simulink library "Power_FuelCell1Motor"  (R2019b)
settings: Solver=VariableStepAuto  StartTime=0.0  StopTime=10.0  RelTol=1e-3
undefined symbols (not defined in the file or in its folder): Init, Powertrain
libraries: fl_lib x84, nesl_utility x29, GasN_lib x21, SimscapeFluids_lib x6, simulink_extras x5, customMath_lib x5, ee_lib x3, gn_supplement_lib x2, simulink x2, custom_dcdc_uni_lib x1, sm_lib x1
(part 1 of 2)
Description:
  | Component of Simscape Vehicle Templates Library
  | 
  | Copyright 2018-2020 The MathWorks, Inc.
settings Model: Creator=smiller  LastModifiedBy=smiller
settings DataIOCC: ReturnWorkspaceOutputs=off
settings DebuggingCC: ArithmeticOperatorsInVariantConditions=warning
settings SFSimCC: CustomCodeUndefinedFunction=UseInterfaceOnly

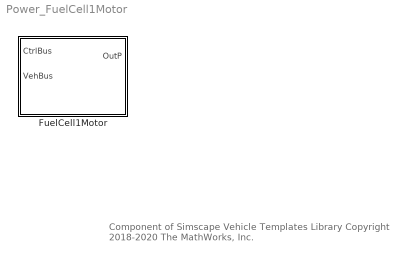
== system Power_FuelCell1Motor ==
  note: Component of Simscape Vehicle Templates Library
      | Copyright 2018-2020 The MathWorks, Inc.
  FuelCell1Motor : Subsystem  mask{Power=Powertrain.Power}
      mask prompts: Power "Power (structure)"
      mask Display: image('sm_car_vehicle_power_fc1motor_IMAGE.png');

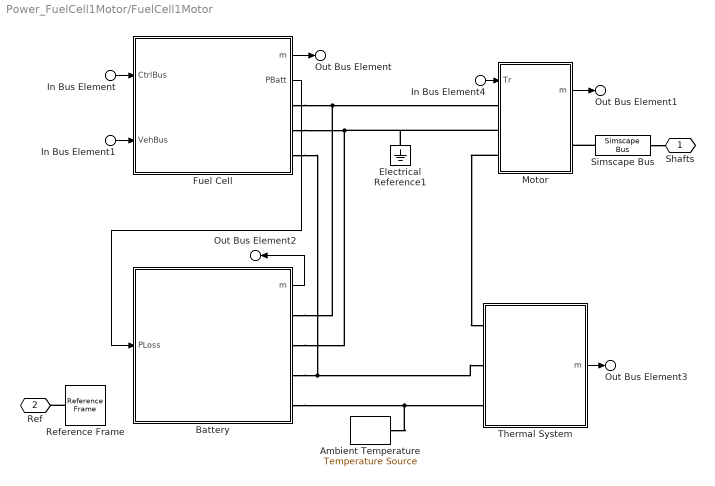
== system Power_FuelCell1Motor/FuelCell1Motor ==
  In Bus Element : Inport  PortName=CtrlBus  Element=FuelCell
  In Bus Element4 : Inport  PortName=CtrlBus  Element=Motor.trqCmd
  In Bus Element1 : Inport  Port=2  PortName=VehBus  Element=Body.CG
  Ambient Temperature : fl_lib/Thermal/Thermal Sources/Temperature Source  temperature=300 K
      settings: SourceProductName=Simscape
  Battery : Subsystem  VariantControl=0  mask{Battery=Power.Battery}
      mask prompts: Battery "Battery (structure)"
      mask Display: image('sm_car_vehicle_power_battery_system_IMAGE.png');
  Electrical Reference1 : fl_lib/Electrical/Electrical Elements/Electrical Reference
  Fuel Cell : Subsystem  VariantControl=0  mask{FuelCell=Power.FuelCell}
      mask prompts: FuelCell "Fuel Cell (structure)"
      mask Display: image('sm_car_vehicle_power_fuel_cell_converter_IMAGE.png');
  Motor : Subsystem  mask{Motor=Power.MotorF}
      mask prompts: Motor "Motor (structure)"
      mask Display: image('sm_car_vehicle_power_emotor_simplified_IMAGE.png');
  Reference Frame : sm_lib/Frames and Transforms/Reference Frame
  Simscape Bus : SimscapeBus  HierarchyStrings=ShaftF
  Thermal System : Subsystem  mask{Cooling=Power.Cooling}
      mask prompts: Cooling "Cooling (structure)"
      mask Display: image('sm_car_vehicle_power_cooling_active1loop_IMAGE.png');
  Shafts : PMIOPort  Side=Left
  Ref : PMIOPort  Port=2  Side=Right
  Out Bus Element : Outport  PortName=OutP  Element=FuelCell
  Out Bus Element1 : Outport  PortName=OutP  Element=Motor
  Out Bus Element2 : Outport  PortName=OutP  Element=Battery
  Out Bus Element3 : Outport  PortName=OutP  Element=Thermal
  wires:
  Fuel Cell/2(PBatt) -> Battery/1(PLoss)
  In Bus Element/1 -> Fuel Cell/1(CtrlBus)
  In Bus Element4/1 -> Motor/1(Tr)
  In Bus Element1/1 -> Fuel Cell/2(VehBus)
  Motor/1(m) -> Out Bus Element1/1
  Fuel Cell/1(m) -> Out Bus Element/1
  Thermal System/1(m) -> Out Bus Element3/1
  Battery/1(m) -> Out Bus Element2/1
  connections:
  Simscape Bus/LConn1 -- Motor/RConn1
  Battery/RConn2 -- Motor/LConn2 -- Electrical Reference1/LConn1 -- Fuel Cell/RConn2
  Simscape Bus/RConn1 -- Shafts/RConn1
  Motor/LConn3 -- Thermal System/LConn1
  Battery/RConn3 -- Fuel Cell/RConn3 -- Thermal System/LConn2
  Ambient Temperature/LConn1 -- Battery/RConn4 -- Thermal System/LConn3
  Battery/RConn1 -- Fuel Cell/RConn1 -- Motor/LConn1
  Reference Frame/RConn1 -- Ref/RConn1

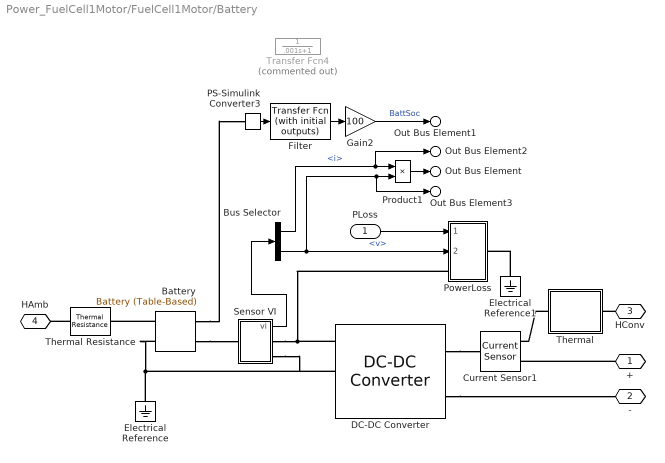
== system Power_FuelCell1Motor/FuelCell1Motor/Battery ==
  PLoss : Inport
  Battery : ee_lib/Sources/Battery (Table-Based)  SOC_vec=Battery.vNoLoad.SOC.Value  T_dependence=ee.enum.temperature_dependence.yes  T_vec=Battery.vNoLoad.T.Value K  V0_mat=Battery.vNoLoad.V0.Value V  V0_vec=[3.1, 3.27, 3.31, 3.5] V  R0_mat=Battery.rTerminal.R0.Value Ohm  R0_vec=[.015, .017, .012, .013] Ohm  AH_vec=Battery.AhTable.Ah.Value hr*A  AH=4.1 hr*A  prm_leak=1  Rleak_vec=ones(size(Battery.vNoLoad.T.Value))*10000 Ohm  Rleak=7e3 Ohm  prm_dyn=1  R1_mat=[.089, .076, .01; .042, .022, .099; .019, .007, .002; .051, .043, .029] Ohm  R1_vec=[.076, .022, .007, .043] Ohm  tau1_mat=[44, 148, 235; 93, 110, 1000; 19, 27, 133; .5, 22, 3] s  tau1_vec=[148, 110, 27, 22] s  R2_mat=[.014, .382, .407; .028, .006, .007; .014, .007, .006; .333, .956, .912] Ohm  R2_vec=[.382, .006, .007, .956] Ohm  tau2_mat=[1, 44, 5644; 11, 24, 506; 2, 14, 330; 3310, 13419, 30216] s  tau2_vec=[44, 24, 14, 13419] s  R3_mat=[.014, .382, .407; .028, .006, .007; .014, .007, .006; .333, .956, .912] Ohm  R3_vec=[.382, .006, .007, .956] Ohm  tau3_mat=[1, 44, 5644; 11, 24, 506; 2, 14, 330; 3310, 13419, 30216] s  tau3_vec=[44, 24, 14, 13419] s  R4_mat=[.014, .382, .407; .028, .006, .007; .014, .007, .006; .333, .956, .912] Ohm  R4_vec=[.382, .006, .007, .956] Ohm  tau4_mat=[1, 44, 5644; 11, 24, 506; 2, 14, 330; 3310, 13419, 30216] s  tau4_vec=[44, 24, 14, 13419] s  R5_mat=[.014, .382, .407; .028, .006, .007; .014, .007, .006; .333, .956, .912] Ohm  R5_vec=[.382, .006, .007, .956] Ohm  tau5_mat=[1, 44, 5644; 11, 24, 506; 2, 14, 330; 3310, 13419, 30216] s  tau5_vec=[44, 24, 14, 13419] s  prm_fade=ee.enum.battery.prm_fade.equations  N0=100  dV0=0  dR0=0  dAH=0  dRleak=0  dR1=0  dR2=0  dR3=0  dR4=0  dR5=0  N0vec=[100, 200, 300]  Tfadevec=[298.15, 323.15] K  dV0vec=[0, 0, 0]  dR0vec=[0, 0, 0]  dAHvec=[0, 0, 0]  dRleakvec=[0, 0, 0]  dR1vec=[0, 0, 0]  dR2vec=[0, 0, 0]  dR3vec=[0, 0, 0]  dR4vec=[0, 0, 0]  dR5vec=[0, 0, 0]  dV0mat=[0, 0; 0, 0; 0, 0]  dR0mat=[0, 0; 0, 0; 0, 0]  dAHmat=[0, 0; 0, 0; 0, 0]  dRleakmat=[0, 0; 0, 0; 0, 0]  dR1mat=[0, 0; 0, 0; 0, 0]  dR2mat=[0, 0; 0, 0; 0, 0]  dR3mat=[0, 0; 0, 0; 0, 0]  dR4mat=[0, 0; 0, 0; 0, 0]  dR5mat=[0, 0; 0, 0; 0, 0]  temperature=Battery.TInit.Value K  i_specify=off  i_priority=None  i=0 A  i_nominal_specify=off  i_nominal_unit=A  i_nominal_value=1  v_specify=off  v_priority=None  v=0 V  v_nominal_specify=off  v_nominal_unit=V  v_nominal_value=1  stateOfCharge_specify=on  stateOfCharge_priority=High  stateOfCharge=Battery.SOCInit.Value  stateOfCharge_nominal_specify=off  stateOfCharge_nominal_unit=1  stateOfCharge_nominal_value=1  num_cycles_specify=off  num_cycles_priority=High  num_cycles=0  num_cycles_nominal_specify=off  num_cycles_nominal_unit=1  num_cycles_nominal_value=1  thermal_mass=Battery.mThermal.Value J/K  temperature_specify=on  temperature_priority=High  temperature_nominal_specify=off  temperature_nominal_unit=K  temperature_nominal_value=1
      settings: SourceProductName=Simscape Electrical  SourceProductBaseCode=PS  InternalSimscapePortConfiguration="{\"Bottom\":[],\"Left\":[{\"id\":\"p\",\"label\":\"+\",\"type\":\"foundation.electrical.electrical\"},{\"id\":\"soc\",\"label\":\"SOC\",\"type\":\"output\"}],\"Right\":[{\"id\":\"n\",\"label\":\"-\",\"type\":\"foundation.electrical.electrical\"},{\"id\":\"H\",\"label\":\"H\",\"type\":\"foundation.thermal.thermal\"}],\"Top\":[]}"
  Bus Selector : BusSelector  OutputSignals=i,v
  Current Sensor1 : fl_lib/Electrical/Electrical Sensors/Current Sensor
  DC-DC Converter : ee_lib/Semiconductors & Converters/Converters/DC-DC Converter  v_ref="Battery.Converter.vRef.Value  V"  P_rated=Battery.Converter.power.Value W  droop_param=1  droop=Battery.Converter.droopVpA.Value V/A  droop_percent=2  reversible=1  efficiency=Battery.Converter.efficiency.Value  P_fixed=Battery.Converter.lossFixed.Value W  model_dynamics=0  tau=0.02 s  v_ini=650 V  G_diode=1e-6 1/Ohm  i1_max=Battery.Converter.iMaxSupply.Value A  fault_condition=1  fault_threshold=0.5  thermal_mass=100 J/K  initial_temperature=298.15 K
      settings: SourceProductName=Simscape Electrical  SourceProductBaseCode=PS  InternalSimscapePortConfiguration="{\"Bottom\":[],\"Left\":[{\"id\":\"p1\",\"label\":\"1+\",\"type\":\"foundation.electrical.electrical\"},{\"id\":\"n1\",\"label\":\"1-\",\"type\":\"foundation.electrical.electrical\"},{\"id\":\"F\",\"label\":\"F\",\"type\":\"input\"}],\"Right\":[{\"id\":\"p2\",\"label\":\"2+\",\"type\":\"foundation.electrical.electrical\"},{\"id\":\"n2\",\"label\":\"2-\",\"type\":\"foundation.electrical.electrical\"}],\"Top\":[]}"
  Electrical Reference : fl_lib/Electrical/Electrical Elements/Electrical Reference
  Electrical Reference1 : fl_lib/Electrical/Electrical Elements/Electrical Reference
  Filter : simulink_extras/Additional Linear/Transfer Fcn (with initial outputs)  N=[1]  D=[.01 1]  Y0=Battery.SOCInit.Value  U0=0
  Gain2 : Gain  Gain=100
  PS-Simulink Converter3 : nesl_utility/PS-Simulink Converter  PhysicalDomain=network_engine_domain  SubClassName=ps_output  LeftPortType=input  RightPortType=output  PseudoPeriodic=off  Frequencies=[]  Unit=1  AffineConversion=off
  PowerLoss : Subsystem
  Product1 : Product
  Sensor VI : Subsystem
  Thermal : Subsystem
  Thermal Resistance : fl_lib/Thermal/Thermal Elements/Thermal Resistance  resistance=Battery.rThermal.Value K/W  T_specify=off  T_priority=None  T=0 K  T_nominal_specify=off  T_nominal_unit=K  T_nominal_value=1  Q_specify=off  Q_priority=None  Q=0 W  Q_nominal_specify=off  Q_nominal_unit=W  Q_nominal_value=1
      settings: SourceProductName=Simscape  SourceProductBaseCode=SS
  Transfer Fcn4 : TransferFcn  Commented=on  Denominator=[.001 1]
  + : PMIOPort  Side=Right
  - : PMIOPort  Port=2  Side=Right
  HConv : PMIOPort  Port=3  Side=Right
  HAmb : PMIOPort  Port=4  Side=Right
  Out Bus Element : Outport  PortName=m  Element=Power
  Out Bus Element1 : Outport  PortName=m  Element=SOC
  Out Bus Element2 : Outport  PortName=m  Element=i
  Out Bus Element3 : Outport  PortName=m  Element=v
  wires:
  PS-Simulink Converter3/1 -> Filter/1
  Gain2/1 -> Out Bus Element1/1  "BattSoc"
  Filter/1 -> Gain2/1
  Bus Selector/2 -> Product1/2, Out Bus Element3/1, PowerLoss/2(VBatt)  "<v>"
  PLoss/1 -> PowerLoss/1(PLoss)
  Bus Selector/1 -> Product1/1, Out Bus Element2/1  "<i>"
  Product1/1 -> Out Bus Element/1
  Sensor VI/1(vi) -> Bus Selector/1
  connections:
  PowerLoss/LConn1 -- DC-DC Converter/LConn1 -- Sensor VI/RConn1
  Battery/LConn2 -- PS-Simulink Converter3/LConn1
  Battery/LConn1 -- Sensor VI/LConn1
  Electrical Reference/LConn1 -- Battery/RConn1 -- DC-DC Converter/LConn2 -- Sensor VI/RConn2
  Battery/RConn2 -- Thermal Resistance/RConn1
  +/RConn1 -- Current Sensor1/RConn2
  DC-DC Converter/RConn2 -- -/RConn1
  DC-DC Converter/RConn1 -- Current Sensor1/LConn1
  Thermal Resistance/LConn1 -- HAmb/RConn1
  Electrical Reference1/LConn1 -- PowerLoss/RConn1
  HConv/RConn1 -- Thermal/RConn1
  Thermal/LConn1 -- Current Sensor1/RConn1

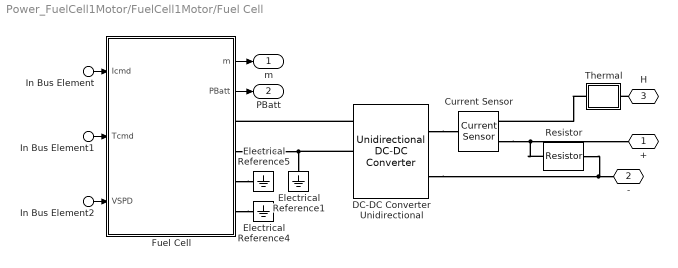
== system Power_FuelCell1Motor/FuelCell1Motor/Fuel Cell ==
  In Bus Element : Inport  PortName=CtrlBus  Element=iCmd
  In Bus Element1 : Inport  PortName=CtrlBus  Element=TFuelCellCmd
  In Bus Element2 : Inport  Port=2  PortName=VehBus  Element=vx
  Current Sensor : fl_lib/Electrical/Electrical Sensors/Current Sensor
  DC-DC Converter Unidirectional : custom_dcdc_uni_lib/Unidirectional DC-DC Converter  v_ref=FuelCell.Converter.vRef.Value V  P_rated=FuelCell.Converter.power.Value W  droop=FuelCell.Converter.droopVpA.Value V/A  efficiency=FuelCell.Converter.efficiency.Value  P_fixed=FuelCell.Converter.lossFixed.Value W  v_ini=650 V  G_diode=1e-6 1/Ohm  i1_max=FuelCell.Converter.iMaxSupply.Value A  fault_threshold=0.5
      settings: InternalSimscapePortConfiguration="{\"Bottom\":[],\"Left\":[{\"id\":\"p1\",\"label\":\"1+\",\"type\":\"foundation.electrical.electrical\"},{\"id\":\"n1\",\"label\":\"1-\",\"type\":\"foundation.electrical.electrical\"},{\"id\":\"F\",\"label\":\"F\",\"type\":\"input\"}],\"Right\":[{\"id\":\"p2\",\"label\":\"2+\",\"type\":\"foundation.electrical.electrical\"},{\"id\":\"n2\",\"label\":\"2-\",\"type\":\"foundation.electrical.electrical\"}],\"Top\":[]}"
  Electrical Reference1 : fl_lib/Electrical/Electrical Elements/Electrical Reference
  Electrical Reference4 : fl_lib/Electrical/Electrical Elements/Electrical Reference
  Electrical Reference5 : fl_lib/Electrical/Electrical Elements/Electrical Reference
  Fuel Cell : Subsystem
      mask Display: image('sm_car_vehicle_power_fuel_cell_IMAGE.png');
  Resistor : fl_lib/Electrical/Electrical Elements/Resistor  R=1e7 Ohm  i_specify=off  i_priority=None  i=0 A  i_nominal_specify=off  i_nominal_unit=A  i_nominal_value=1  v_specify=off  v_priority=None  v=0 V  v_nominal_specify=off  v_nominal_unit=V  v_nominal_value=1
  Thermal : Subsystem
  + : PMIOPort  Side=Right
  - : PMIOPort  Port=2  Side=Right
  H : PMIOPort  Port=3  Side=Right
  m : Outport
  PBatt : Outport  Port=2
  wires:
  In Bus Element2/1 -> Fuel Cell/3(VSPD)
  In Bus Element1/1 -> Fuel Cell/2(Tcmd)
  In Bus Element/1 -> Fuel Cell/1(Icmd)
  Fuel Cell/1(m) -> m/1
  Fuel Cell/2(PBatt) -> PBatt/1
  connections:
  Fuel Cell/RConn2 -- DC-DC Converter Unidirectional/LConn2 -- Electrical Reference1/LConn1
  Resistor/RConn1 -- DC-DC Converter Unidirectional/RConn2 -- -/RConn1
  Current Sensor/RConn2 -- Resistor/LConn1 -- +/RConn1
  Fuel Cell/RConn3 -- Electrical Reference5/LConn1
  Fuel Cell/RConn4 -- Electrical Reference4/LConn1
  DC-DC Converter Unidirectional/LConn1 -- Fuel Cell/RConn1
  DC-DC Converter Unidirectional/RConn1 -- Current Sensor/LConn1
  H/RConn1 -- Thermal/RConn1
  Thermal/LConn1 -- Current Sensor/RConn1

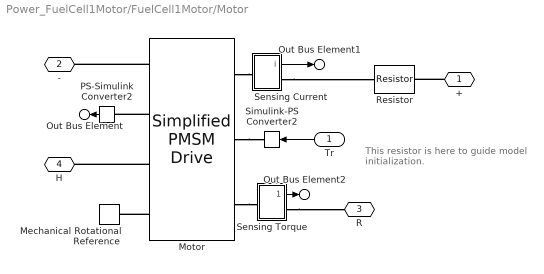
== system Power_FuelCell1Motor/FuelCell1Motor/Motor ==
  note: This resistor is here to guide model initialization.
  Tr : Inport
  Mechanical Rotational Reference : fl_lib/Mechanical/Rotational Elements/Mechanical Rotational Reference
  Motor : ee_lib/Electromechanical/Permanent Magnet/Simplified PMSM Drive  torque_speed_param=1  w_t=Motor.TorqueSpd.w.Value rpm  T_t=Motor.TorqueSpd.trq.Value N*m  torque_max=0.1 N*m  power_max=30 W  Tc=1/Motor.fActuatorCutoff.Value s  losses_param=3  eff=100  w_eff=3750 rpm  T_eff=0.08 N*m  Piron=0 W  Pbase=0 W  w_eff_vec=Motor.TorqueSpd.w.Value rpm  T_eff_vec=Motor.LossTable.trq.Value N*m  v_eff_vec=[100, 250, 400] V  losses_mat=[1.49, 1.67, 2.21, 3.1; .42, .69, 1.14, 2.03; .06, .24, .78, 1.68; .42, .69, 1.14, 2.03; 1.49, 1.67, 2.21, 3.1] W  efficiency_mat=Motor.LossTable.efficiency.Value  losses_mat_3D=ones(5, 4, 3) W  efficiency_mat_3D=95 * ones(5, 4, 3)  Res=Motor.Rsupply.Value Ohm  J=Motor.J.Value kg*m^2  lam=Motor.b.Value N*m/(rad/s)  speed0=0 rpm  faulted_specify=off  faulted_priority=None  faulted=0  faulted_nominal_specify=off  faulted_nominal_unit=1  faulted_nominal_value=1  alpha=3.93e-3 1/K  Tmeas=Motor.ThermalLoss.T1.Value degC  Tmeas2=Motor.ThermalLoss.T2.Value degC  losses_mat_T2=[1.49, 1.74, 2.49, 3.74; .42, .67, 1.42, 2.67; .06, .31, 1.06, 2.31; .42, .67, 1.42, 2.67; 1.49, 1.74, 2.49, 3.74] W  efficiency_mat_T2=Motor.ThermalLoss.efficiency.Value  losses_mat_3D_T2=ones(5, 4, 3) W  efficiency_mat_3D_T2=95 * ones(5, 4, 3)  thermal_mass=Motor.ThermalLoss.mThermal.Value J/K  initial_temperature=Motor.ThermalLoss.Tinit.Value K  fault_condition=1  fault_threshold=0.5
      settings: SourceProductName=Simscape Electrical  SourceProductBaseCode=PS  InternalSimscapePortConfiguration="{\"Bottom\":[],\"Left\":[{\"id\":\"Vp\",\"label\":\"+\",\"type\":\"foundation.electrical.electrical\"},{\"id\":\"Tr\",\"label\":\"Tr\",\"type\":\"input\"},{\"id\":\"R\",\"label\":\"R\",\"type\":\"foundation.mechanical.rotational.rotational\"}],\"Right\":[{\"id\":\"Vm\",\"label\":\"-\",\"type\":\"foundation.electrical.electrical\"},{\"id\":\"Omega\",\"label\":\"w\",\"type\":\"output\"},{\"id\":\"H\",\"label\":\"H\",\"type\":\"foundation.thermal.thermal\"},{\"id\":\"C\",\"label\":\"C\",\"type\":\"foundation.mechanical.rotational.rotational\"}],\"Top\":[]}"
  PS-Simulink Converter2 : nesl_utility/PS-Simulink Converter  PhysicalDomain=network_engine_domain  SubClassName=ps_output  LeftPortType=input  RightPortType=output  PseudoPeriodic=off  Frequencies=[]  Unit=rad/s  AffineConversion=off
  Resistor : fl_lib/Electrical/Electrical Elements/Resistor  R=1e-6 Ohm  i_specify=on  i_priority=High  i=0.1*Init.Front.nWheel.Value(1) A  i_nominal_specify=off  i_nominal_unit=A  i_nominal_value=1  v_specify=off  v_priority=None  v=0 V  v_nominal_specify=off  v_nominal_unit=V  v_nominal_value=1
  Sensing Current : Subsystem
  Sensing Torque : Subsystem
  Simulink-PS Converter2 : nesl_utility/Simulink-PS Converter  PhysicalDomain=network_engine_domain  SubClassName=ps_input  LeftPortType=input  RightPortType=output  PseudoPeriodic=off  Frequencies=[]  NoiseDistribution=none  NoiseParameters=[]  Unit=N*m  AffineConversion=off  FilteringAndDerivatives=provide  SimscapeFilterOrder=1  InputFilterTimeConstant=0.001  UdotUserProvided=0
  + : PMIOPort  Side=Left
  - : PMIOPort  Port=2  Side=Left
  R : PMIOPort  Port=3  Side=Right
  H : PMIOPort  Port=4  Side=Left
  Out Bus Element : Outport  PortName=m  Element=w
  Out Bus Element1 : Outport  PortName=m  Element=i
  Out Bus Element2 : Outport  PortName=m  Element=trq
  wires:
  PS-Simulink Converter2/1 -> Out Bus Element/1
  Tr/1 -> Simulink-PS Converter2/1
  Sensing Current/1(i) -> Out Bus Element1/1
  Sensing Torque/1(trq) -> Out Bus Element2/1
  connections:
  Motor/RConn4 -- Mechanical Rotational Reference/LConn1
  Motor/LConn2 -- Simulink-PS Converter2/RConn1
  Motor/LConn3 -- Sensing Torque/LConn1
  Motor/LConn1 -- Sensing Current/LConn1
  Motor/RConn1 -- -/RConn1
  Motor/RConn3 -- H/RConn1
  Motor/RConn2 -- PS-Simulink Converter2/LConn1
  Sensing Current/RConn1 -- Resistor/LConn1
  Sensing Torque/RConn1 -- R/RConn1
  +/RConn1 -- Resistor/RConn1

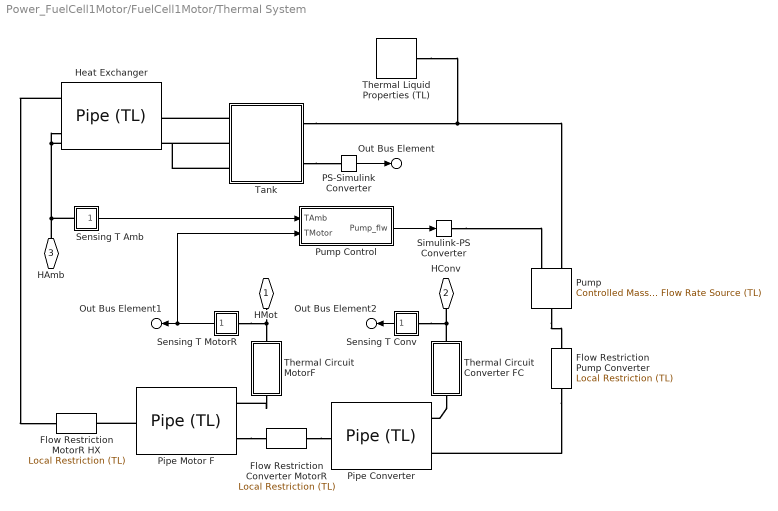
== system Power_FuelCell1Motor/FuelCell1Motor/Thermal System ==
  Flow Restriction Converter MotorR : fl_lib/Thermal Liquid/Elements/Local Restriction (TL)  restriction_type=foundation.enum.restriction_type.fixed  restriction_area=Cooling.Restriction.area.Value m^2  min_area=1e-10 m^2  max_area=0.005 m^2  area=Cooling.Restriction.areaPorts.Value m^2  Cd=Cooling.Restriction.dischargeCoeff.Value  pressure_recovery=simscape.enum.onoff.on  Re_c=Cooling.Restriction.CriticalReynolds.Value
      settings: SourceProductName=Simscape  SourceProductBaseCode=SS
  Flow Restriction MotorR HX : fl_lib/Thermal Liquid/Elements/Local Restriction (TL)  restriction_type=foundation.enum.restriction_type.fixed  restriction_area=Cooling.Restriction.area.Value m^2  min_area=1e-10 m^2  max_area=0.005 m^2  area=Cooling.Restriction.areaPorts.Value m^2  Cd=Cooling.Restriction.dischargeCoeff.Value  pressure_recovery=simscape.enum.onoff.on  Re_c=Cooling.Restriction.CriticalReynolds.Value
      settings: SourceProductName=Simscape  SourceProductBaseCode=SS
  Flow Restriction Pump Converter : fl_lib/Thermal Liquid/Elements/Local Restriction (TL)  restriction_type=foundation.enum.restriction_type.fixed  restriction_area=Cooling.Restriction.area.Value m^2  min_area=1e-10 m^2  max_area=0.005 m^2  area=Cooling.Restriction.areaPorts.Value m^2  Cd=Cooling.Restriction.dischargeCoeff.Value  pressure_recovery=simscape.enum.onoff.on  Re_c=Cooling.Restriction.CriticalReynolds.Value
      settings: SourceProductName=Simscape  SourceProductBaseCode=SS
  Heat Exchanger : SimscapeFluids_lib/Thermal Liquid/Pipes & Fittings/Pipe (TL)  dynamic_compressibility=0  inertia=0  num_segments=1  pipe_length=Cooling.HX.x.Value m  area=Cooling.HX.area.Value m^2  Dh=Cooling.HX.diameter.Value m  wall_spec=1  Dh_rigid=0.01 m  wall_compliance=1.2e-6 m/MPa  wall_time_constant=0.01 s  elevation_gain=Cooling.HX.elevation.Value m  g=9.81 m/s^2  pressure_loss_spec=1  length_add=Cooling.HX.xResistance.Value m  roughness=Cooling.HX.roughness.Value m  Re_friction_TLU=[ 400 1000 1.5e+3 3e+3 4e+3 6e+3 1e+4 2e+4 4e+4 6e+4 1e+5 1e+8 ]  friction_factor_TLU=[ 0.264 0.112 0.07099999999999999 0.0417 0.0387 0.0268 0.025 0.0232 0.0226 0.022 0.0214 0.0214 ]  shape_factor=Cooling.HX.frictionDarcy.Value  mdot_nominal=[ 0.1 1 ] kg/s  p_diff_nominal=[ 0.001 0.01 ] MPa  mdot_threshold=1e-6 kg/s  Re_lam=Cooling.HX.laminarReynoldsMax.Value  Re_tur=Cooling.HX.turbulentReynoldsMin.Value  heat_transfer_spec=1  mdot_nominal_heat=[ 0.1 1 ] kg/s  T_in_nominal=[ 293.15 293.15 ] K  T_out_nominal=[ 300 300 ] K  p_in_nominal_heat=[ 0.101325 0.101325 ] MPa  T_wall_nominal=[ 303.15 303.15 ] K  a_coeff=0.023  b_Re_power=0.8  c_Pr_power=0.4  Nu_lam=Cooling.HX.laminarNusselt.Value  Re_Colburn_TLU=[ 100 150 1000 ]  Colburn_factor_TLU=[ 0.019 0.013 0.002 ]  Re_Nu_TLU=[ 100 150 1000 ]  Pr_Nu_TLU=[ 1 10 ]  Nu_TLU=[ 3.72 4.21; 3.75 4.44; 4.21 7.15 ]  T0_vec=300 K  p0_vec=0.101325 MPa  mdot0=0.1 kg/s
      settings: SourceProductName=Simscape Fluids  SourceProductBaseCode=SH
  PS-Simulink Converter : nesl_utility/PS-Simulink Converter  PhysicalDomain=network_engine_domain  SubClassName=ps_output  LeftPortType=input  RightPortType=output  PseudoPeriodic=off  Frequencies=[]  Unit=K  AffineConversion=off
  Pipe Converter : SimscapeFluids_lib/Thermal Liquid/Pipes & Fittings/Pipe (TL)  dynamic_compressibility=0  inertia=0  num_segments=1  pipe_length=Cooling.Converter.Pipe.x.Value m  area="Cooling.Converter.Pipe.area.Value  m^2"  Dh=Cooling.Converter.Pipe.diameter.Value m  wall_spec=1  Dh_rigid=0.01 m  wall_compliance=1.2e-6 m/MPa  wall_time_constant=0.01 s  elevation_gain=Cooling.Converter.Pipe.elevation.Value m  g=9.81 m/s^2  pressure_loss_spec=1  length_add=Cooling.Converter.Pipe.xResistance.Value m  roughness=Cooling.Converter.Pipe.roughness.Value m  Re_friction_TLU=[ 400 1000 1.5e+3 3e+3 4e+3 6e+3 1e+4 2e+4 4e+4 6e+4 1e+5 1e+8 ]  friction_factor_TLU=[ 0.264 0.112 0.07099999999999999 0.0417 0.0387 0.0268 0.025 0.0232 0.0226 0.022 0.0214 0.0214 ]  shape_factor=Cooling.Converter.Pipe.frictionDarcy.Value  mdot_nominal=[ 0.1 1 ] kg/s  p_diff_nominal=[ 0.001 0.01 ] MPa  mdot_threshold=1e-6 kg/s  Re_lam=Cooling.Converter.Pipe.laminarReynoldsMax.Value  Re_tur=Cooling.Converter.Pipe.turbulentReynoldsMin.Value  heat_transfer_spec=1  mdot_nominal_heat=[ 0.1 1 ] kg/s  T_in_nominal=[ 293.15 293.15 ] K  T_out_nominal=[ 300 300 ] K  p_in_nominal_heat=[ 0.101325 0.101325 ] MPa  T_wall_nominal=[ 303.15 303.15 ] K  a_coeff=0.023  b_Re_power=0.8  c_Pr_power=0.4  Nu_lam=Cooling.Converter.Pipe.laminarNusselt.Value  Re_Colburn_TLU=[ 100 150 1000 ]  Colburn_factor_TLU=[ 0.019 0.013 0.002 ]  Re_Nu_TLU=[ 100 150 1000 ]  Pr_Nu_TLU=[ 1 10 ]  Nu_TLU=[ 3.72 4.21; 3.75 4.44; 4.21 7.15 ]  T0_vec=300 K  p0_vec=0.101325 MPa  mdot0=0.1 kg/s
      settings: SourceProductName=Simscape Fluids  SourceProductBaseCode=SH
  Pipe Motor F : SimscapeFluids_lib/Thermal Liquid/Pipes & Fittings/Pipe (TL)  dynamic_compressibility=0  inertia=0  num_segments=1  pipe_length=Cooling.MotorF.Pipe.x.Value m  area=Cooling.MotorF.Pipe.area.Value m^2  Dh=Cooling.MotorF.Pipe.diameter.Value m  wall_spec=1  Dh_rigid=0.01 m  wall_compliance=1.2e-6 m/MPa  wall_time_constant=0.01 s  elevation_gain=Cooling.MotorF.Pipe.elevation.Value m  g=9.81 m/s^2  pressure_loss_spec=1  length_add=Cooling.MotorF.Pipe.xResistance.Value m  roughness=Cooling.MotorF.Pipe.roughness.Value m  Re_friction_TLU=[ 400 1000 1.5e+3 3e+3 4e+3 6e+3 1e+4 2e+4 4e+4 6e+4 1e+5 1e+8 ]  friction_factor_TLU=[ 0.264 0.112 0.07099999999999999 0.0417 0.0387 0.0268 0.025 0.0232 0.0226 0.022 0.0214 0.0214 ]  shape_factor=Cooling.MotorF.Pipe.frictionDarcy.Value  mdot_nominal=[ 0.1 1 ] kg/s  p_diff_nominal=[ 0.001 0.01 ] MPa  mdot_threshold=1e-6 kg/s  Re_lam=Cooling.MotorF.Pipe.laminarReynoldsMax.Value  Re_tur=Cooling.MotorF.Pipe.turbulentReynoldsMin.Value  heat_transfer_spec=1  mdot_nominal_heat=[ 0.1 1 ] kg/s  T_in_nominal=[ 293.15 293.15 ] K  T_out_nominal=[ 300 300 ] K  p_in_nominal_heat=[ 0.101325 0.101325 ] MPa  T_wall_nominal=[ 303.15 303.15 ] K  a_coeff=0.023  b_Re_power=0.8  c_Pr_power=0.4  Nu_lam=Cooling.MotorF.Pipe.laminarNusselt.Value  Re_Colburn_TLU=[ 100 150 1000 ]  Colburn_factor_TLU=[ 0.019 0.013 0.002 ]  Re_Nu_TLU=[ 100 150 1000 ]  Pr_Nu_TLU=[ 1 10 ]  Nu_TLU=[ 3.72 4.21; 3.75 4.44; 4.21 7.15 ]  T0_vec=300 K  p0_vec=0.101325 MPa  mdot0=0.1 kg/s
      settings: SourceProductName=Simscape Fluids  SourceProductBaseCode=SH
  Pump : fl_lib/Thermal Liquid/Sources/Controlled Mass Flow Rate Source (TL)  area=Cooling.Pump.area.Value m^2
      settings: SourceProductName=Simscape  SourceProductBaseCode=SS  InternalSimscapePortConfiguration="{\"Bottom\":[],\"Left\":[{\"id\":\"A\",\"label\":\"A\",\"type\":\"foundation.thermal_liquid.thermal_liquid\"},{\"id\":\"M\",\"label\":\"M\",\"type\":\"input\"}],\"Right\":[{\"id\":\"B\",\"label\":\"B\",\"type\":\"foundation.thermal_liquid.thermal_liquid\"}],\"Top\":[]}"
  Pump Control : Subsystem
  Sensing T Amb : Subsystem
  Sensing T Conv : Subsystem
  Sensing T MotorR : Subsystem
  Simulink-PS Converter : nesl_utility/Simulink-PS Converter  PhysicalDomain=network_engine_domain  SubClassName=ps_input  LeftPortType=input  RightPortType=output  PseudoPeriodic=off  Frequencies=[]  NoiseDistribution=none  NoiseParameters=[]  Unit=kg/s  AffineConversion=off  FilteringAndDerivatives=filter  SimscapeFilterOrder=1  InputFilterTimeConstant=1  UdotUserProvided=0
  Tank : Subsystem
  Thermal Circuit Converter FC : Subsystem
  Thermal Circuit MotorF : Subsystem
  Thermal Liquid Properties (TL) : SimscapeFluids_lib/Thermal Liquid/Utilities/Thermal Liquid Properties (TL)  fluid_list=fluids.thermal_liquid.utilities.enum.thermal_liquid_fluid_list.ethylene_glycol  concentration_param_EG=fluids.thermal_liquid.utilities.enum.thermal_liquid_concentration.volume_fraction  concentration_param_PG=fluids.thermal_liquid.utilities.enum.thermal_liquid_concentration.volume_fraction  c_mass_SW=3.5e-3  c_mass_EG=0.1  c_mass_PG=0.1  c_mass_GL=0.1  c_vol_EG=Cooling.Fluid.rEthyleneGlycol.Value  c_vol_PG=0.1  beta_const_EG=Cooling.Fluid.bulkModulus.Value GPa  beta_const_PG=2.1791 GPa  beta_const_GL=2.1791 GPa  p_min_EG=Cooling.Fluid.pMin.Value MPa  p_min_PG=0.01 MPa  p_min_GL=0.01 MPa  p_max_EG=Cooling.Fluid.pMax.Value MPa  p_max_PG=50 MPa  p_max_GL=50 MPa  p_atm=0.101325 MPa
      settings: SourceProductName=Simscape Fluids  SourceProductBaseCode=SH
  HMot : PMIOPort  Side=Left
  HConv : PMIOPort  Port=2  Side=Left
  HAmb : PMIOPort  Port=3  Side=Left
  Out Bus Element : Outport  PortName=m  Element=TCoolant
  Out Bus Element1 : Outport  PortName=m  Element=TMotorF
  Out Bus Element2 : Outport  PortName=m  Element=TConverter
  wires:
  Pump Control/1(Pump_flw) -> Simulink-PS Converter/1
  PS-Simulink Converter/1 -> Out Bus Element/1
  Sensing T MotorR/1(T) -> Pump Control/2(TMotor), Out Bus Element1/1
  Sensing T Amb/1(T) -> Pump Control/1(TAmb)
  Sensing T Conv/1(T) -> Out Bus Element2/1
  connections:
  Pipe Motor F/LConn1 -- Flow Restriction Converter MotorR/RConn1
  Flow Restriction Converter MotorR/LConn1 -- Pipe Converter/RConn1
  Pump/RConn1 -- Flow Restriction Pump Converter/LConn1
  Simulink-PS Converter/RConn1 -- Pump/LConn2
  Thermal Circuit MotorF/RConn1 -- Pipe Motor F/LConn2
  HAmb/RConn1 -- Sensing T Amb/LConn1 -- Tank/LConn3 -- Tank/LConn2 -- Heat Exchanger/LConn2
  Heat Exchanger/LConn1 -- Flow Restriction MotorR HX/RConn1
  Flow Restriction Pump Converter/RConn1 -- Pipe Converter/LConn1
  Pipe Motor F/RConn1 -- Flow Restriction MotorR HX/LConn1
  Tank/LConn1 -- Heat Exchanger/RConn1
  Tank/RConn1 -- Thermal Liquid Properties (TL)/RConn1 -- Pump/LConn1
  Thermal Circuit Converter FC/RConn1 -- Pipe Converter/LConn2
  HMot/RConn1 -- Thermal Circuit MotorF/LConn1 -- Sensing T MotorR/LConn1
  Tank/RConn2 -- PS-Simulink Converter/LConn1
  Thermal Circuit Converter FC/LConn1 -- Sensing T Conv/LConn1 -- HConv/RConn1

== system Power_FuelCell1Motor/FuelCell1Motor/Battery/PowerLoss ==
  PLoss : Inport
  VBatt : Inport  Port=2
  Controlled Current Source : fl_lib/Electrical/Electrical Sources/Controlled Current Source
  Divide : Product  Inputs=*/
  Saturation : Saturate  UpperLimit=inf  LowerLimit=200
  Simulink-PS Converter : nesl_utility/Simulink-PS Converter  PhysicalDomain=network_engine_domain  SubClassName=ps_input  LeftPortType=input  RightPortType=output  PseudoPeriodic=off  Frequencies=[]  NoiseDistribution=none  NoiseParameters=[]  Unit=A  AffineConversion=off  FilteringAndDerivatives=filter  SimscapeFilterOrder=1  InputFilterTimeConstant=0.001  UdotUserProvided=0
  + : PMIOPort  Side=Left
  - : PMIOPort  Port=2  Side=Right
  wires:
  VBatt/1 -> Saturation/1
  PLoss/1 -> Divide/1
  Divide/1 -> Simulink-PS Converter/1
  Saturation/1 -> Divide/2
  connections:
  -/RConn1 -- Controlled Current Source/LConn1
  +/RConn1 -- Controlled Current Source/RConn2
  Simulink-PS Converter/RConn1 -- Controlled Current Source/RConn1

== system Power_FuelCell1Motor/FuelCell1Motor/Battery/Sensor VI ==
  Bus Creator : BusCreator  Inputs=2
  Current Sensor : fl_lib/Electrical/Electrical Sensors/Current Sensor
  PS-Simulink Converter2 : nesl_utility/PS-Simulink Converter  PhysicalDomain=network_engine_domain  SubClassName=ps_output  LeftPortType=input  RightPortType=output  PseudoPeriodic=off  Frequencies=[]  Unit=1  AffineConversion=off
  PS-Simulink Converter4 : nesl_utility/PS-Simulink Converter  PhysicalDomain=network_engine_domain  SubClassName=ps_output  LeftPortType=input  RightPortType=output  PseudoPeriodic=off  Frequencies=[]  Unit=1  AffineConversion=off
  Transfer Fcn1 : TransferFcn  Denominator=[.001 1]
  Transfer Fcn5 : TransferFcn  Denominator=[.001 1]
  Voltage Sensor2 : fl_lib/Electrical/Electrical Sensors/Voltage Sensor
  + : PMIOPort  Side=Left
  - : PMIOPort  Port=2  Side=Right
  G : PMIOPort  Port=3  Side=Right
  vi : Outport
  wires:
  PS-Simulink Converter4/1 -> Transfer Fcn5/1
  PS-Simulink Converter2/1 -> Transfer Fcn1/1
  Transfer Fcn1/1 -> Bus Creator/2  "i"
  Transfer Fcn5/1 -> Bus Creator/1  "v"
  Bus Creator/1 -> vi/1
  connections:
  +/RConn1 -- Current Sensor/LConn1 -- Voltage Sensor2/LConn1
  PS-Simulink Converter4/LConn1 -- Voltage Sensor2/RConn1
  Current Sensor/RConn2 -- -/RConn1
  Voltage Sensor2/RConn2 -- G/RConn1
  Current Sensor/RConn1 -- PS-Simulink Converter2/LConn1

== system Power_FuelCell1Motor/FuelCell1Motor/Battery/Thermal ==
  Controlled Heat Flow Rate Source : fl_lib/Thermal/Thermal Sources/Controlled Heat Flow Rate Source
      settings: SourceProductName=Simscape
  PS Gain : fl_lib/Physical Signals/Functions/PS Gain  Commented=on  gain=0.001 Ohm
  PS Math Function : fl_lib/Physical Signals/Functions/PS Math Function  Commented=on  fcn_choice=foundation.enum.math_function.square
      settings: SourceProductName=Simscape  SourceProductBaseCode=SS
  PS Power Function : customMath_lib/PS Power Function  resistance=Battery.Converter.resistance.Value Ohm
      settings: InternalSimscapePortConfiguration="{\"Bottom\":[],\"Left\":[{\"id\":\"I\",\"label\":\"\",\"type\":\"input\"}],\"Right\":[{\"id\":\"O\",\"label\":\"\",\"type\":\"output\"}],\"Top\":[]}"
  Thermal Mass : fl_lib/Thermal/Thermal Elements/Thermal Mass  mass=Battery.Converter.mThermal.Value kg  sp_heat="Battery.Converter.Cp.Value  J/kg/K"  T_specify=off  T_priority=High  T=300 K  T_nominal_specify=off  T_nominal_unit=K  T_nominal_value=1  Q_specify=off  Q_priority=None  Q=0 W  Q_nominal_specify=off  Q_nominal_unit=W  Q_nominal_value=1
  Thermal Resistance : fl_lib/Thermal/Thermal Elements/Thermal Resistance  resistance=Battery.Converter.rThermal.Value K/W  T_specify=off  T_priority=None  T=0 K  T_nominal_specify=off  T_nominal_unit=K  T_nominal_value=1  Q_specify=off  Q_priority=None  Q=0 W  Q_nominal_specify=off  Q_nominal_unit=W  Q_nominal_value=1
      settings: SourceProductName=Simscape  SourceProductBaseCode=SS
  Thermal Reference3 : fl_lib/Thermal/Thermal Elements/Thermal Reference
  H : PMIOPort  Side=Right
  i : PMIOPort  Port=2  Side=Left
  connections:
  Thermal Resistance/LConn1 -- Thermal Mass/LConn1 -- Controlled Heat Flow Rate Source/LConn1
  PS Gain/LConn1 -- PS Math Function/RConn1
  Thermal Reference3/LConn1 -- Controlled Heat Flow Rate Source/RConn2
  H/RConn1 -- Thermal Resistance/RConn1
  PS Power Function/LConn1 -- i/RConn1
  PS Power Function/RConn1 -- Controlled Heat Flow Rate Source/RConn1

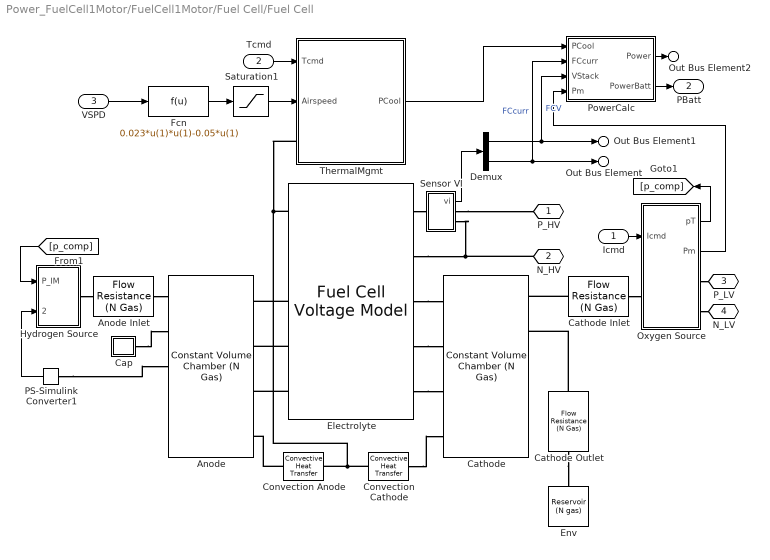
== system Power_FuelCell1Motor/FuelCell1Motor/Fuel Cell/Fuel Cell ==
  Icmd : Inport
  Tcmd : Inport  Port=2
  VSPD : Inport  Port=3
  Anode : GasN_lib/Constant Volume Chamber (N Gas)  V0=FuelCell.Anode.volume.Value m^3  p0=FuelCell.Anode.p.Value MPa  T0=FuelCell.Anode.T.Value degC  comp=GasN.composition_enum.mole  y0=FuelCell.Anode.rMoleFractions.Value'  x0=[1; 0; 0; 0]  tau_c=FuelCell.Anode.timeCondensation.Value s  is_cond=FuelCell.Anode.speciesCondensed.Value'  out_comp=GasN.composition_enum.mass  area_A=FuelCell.Anode.areaPort.Value cm^2  area_B=FuelCell.Anode.areaPort.Value cm^2  area_C=FuelCell.Anode.areaPort.Value cm^2
      settings: InternalSimscapePortConfiguration="{\"Bottom\":[],\"Left\":[{\"id\":\"A\",\"label\":\"A\",\"type\":\"GasN.GasN\"},{\"id\":\"MIn\",\"label\":\"MIn\",\"type\":\"input\"},{\"id\":\"TIn\",\"label\":\"TIn\",\"type\":\"input\"},{\"id\":\"H\",\"label\":\"H\",\"type\":\"foundation.thermal.thermal\"}],\"Right\":[{\"id\":\"B\",\"label\":\"B\",\"type\":\"GasN.GasN\"},{\"id\":\"C\",\"label\":\"C\",\"type\":\"GasN.GasN\"},{\"id\":\"pC\",\"label\":\"p\",\"type\":\"output\"},{\"id\":\"TC\",\"label\":\"T\",\"type\":\"output\"},{\"id\":\"xC_i\",\"label\":\"x_i\",\"type\":\"output\"}],\"Top\":[]}"
  Anode Inlet : GasN_lib/Flow Resistance (N Gas)  var_res=false  delta_p_nominal="FuelCell.AnodeInlet.pDropNominal.Value  MPa"  mdot_nominal=FuelCell.AnodeInlet.mdotNominal.Value kg/s  rho_nominal="FuelCell.AnodeInlet.rhoNominal.Value  kg/m^3"  laminar_fraction=FuelCell.AnodeInlet.rmdotLaminar.Value  area=FuelCell.AnodeInlet.areaPort.Value cm^2  leak_thresh=FuelCell.AnodeInlet.leakageThreshold.Value
      settings: InternalSimscapePortConfiguration="{\"Bottom\":[],\"Left\":[{\"id\":\"A\",\"label\":\"A\",\"type\":\"GasN.GasN\"}],\"Right\":[{\"id\":\"B\",\"label\":\"B\",\"type\":\"GasN.GasN\"}],\"Top\":[]}"
  Cap : Subsystem
  Cathode : GasN_lib/Constant Volume Chamber (N Gas)  V0=FuelCell.Cathode.volume.Value m^3  p0=FuelCell.Cathode.p.Value MPa  T0=FuelCell.Cathode.T.Value degC  comp=GasN.composition_enum.mole  y0=FuelCell.Cathode.rMoleFractions.Value'  x0=[1; 0; 0; 0]  tau_c=FuelCell.Cathode.timeCondensation.Value s  is_cond=FuelCell.Cathode.speciesCondensed.Value'  out_comp=GasN.composition_enum.mass  area_A=FuelCell.Cathode.areaPort.Value cm^2  area_B=FuelCell.Cathode.areaPort.Value cm^2  area_C=FuelCell.Cathode.areaPort.Value cm^2
      settings: InternalSimscapePortConfiguration="{\"Bottom\":[],\"Left\":[{\"id\":\"A\",\"label\":\"A\",\"type\":\"GasN.GasN\"},{\"id\":\"MIn\",\"label\":\"MIn\",\"type\":\"input\"},{\"id\":\"TIn\",\"label\":\"TIn\",\"type\":\"input\"},{\"id\":\"H\",\"label\":\"H\",\"type\":\"foundation.thermal.thermal\"}],\"Right\":[{\"id\":\"B\",\"label\":\"B\",\"type\":\"GasN.GasN\"},{\"id\":\"C\",\"label\":\"C\",\"type\":\"GasN.GasN\"},{\"id\":\"pC\",\"label\":\"p\",\"type\":\"output\"},{\"id\":\"TC\",\"label\":\"T\",\"type\":\"output\"},{\"id\":\"xC_i\",\"label\":\"x_i\",\"type\":\"output\"}],\"Top\":[]}"
  Cathode Inlet : GasN_lib/Flow Resistance (N Gas)  var_res=false  delta_p_nominal=FuelCell.CathodeInlet.pDropNominal.Value MPa  mdot_nominal=FuelCell.CathodeInlet.mdotNominal.Value kg/s  rho_nominal="FuelCell.CathodeInlet.rhoNominal.Value  kg/m^3"  laminar_fraction=FuelCell.CathodeInlet.rmdotLaminar.Value  area=FuelCell.CathodeInlet.areaPort.Value cm^2  leak_thresh=FuelCell.CathodeInlet.leakageThreshold.Value
      settings: InternalSimscapePortConfiguration="{\"Bottom\":[],\"Left\":[{\"id\":\"A\",\"label\":\"A\",\"type\":\"GasN.GasN\"}],\"Right\":[{\"id\":\"B\",\"label\":\"B\",\"type\":\"GasN.GasN\"}],\"Top\":[]}"
  Cathode Outlet : GasN_lib/Flow Resistance (N Gas)  var_res=false  delta_p_nominal=FuelCell.CathodeOutlet.pDropNominal.Value MPa  mdot_nominal=FuelCell.CathodeOutlet.mdotNominal.Value kg/s  rho_nominal=FuelCell.CathodeOutlet.rhoNominal.Value kg/m^3  laminar_fraction=FuelCell.CathodeOutlet.rmdotLaminar.Value  area=FuelCell.CathodeOutlet.areaPort.Value cm^2  leak_thresh=FuelCell.CathodeOutlet.leakageThreshold.Value
      settings: InternalSimscapePortConfiguration="{\"Bottom\":[],\"Left\":[{\"id\":\"A\",\"label\":\"A\",\"type\":\"GasN.GasN\"}],\"Right\":[{\"id\":\"B\",\"label\":\"B\",\"type\":\"GasN.GasN\"}],\"Top\":[]}"
  Convection Anode : fl_lib/Thermal/Thermal Elements/Convective Heat Transfer  area=280*400/8 cm^2  heat_tr_coeff=10 W/(m^2 * K)  T_specify=off  T_priority=None  T=0 K  T_nominal_specify=off  T_nominal_unit=K  T_nominal_value=1  Q_specify=off  Q_priority=None  Q=0 W  Q_nominal_specify=off  Q_nominal_unit=W  Q_nominal_value=1
  Convection Cathode : fl_lib/Thermal/Thermal Elements/Convective Heat Transfer  area=280*400/8 cm^2  heat_tr_coeff=10 W/(m^2 * K)  T_specify=off  T_priority=None  T=0 K  T_nominal_specify=off  T_nominal_unit=K  T_nominal_value=1  Q_specify=off  Q_priority=None  Q=0 W  Q_nominal_specify=off  Q_nominal_unit=W  Q_nominal_value=1
  Demux : Demux  Outputs=2
  Electrolyte : gn_supplement_lib/fuel_cell/Fuel Cell Voltage Model  Ncell=FuelCell.Electrolyte.numCells.Value  Acell=FuelCell.Electrolyte.areaCell.Value cm^2  tcell=FuelCell.Electrolyte.thicknessMembrane.Value cm  io=FuelCell.Electrolyte.exchangeCurrentDensity.Value A/cm^2  iL=FuelCell.Electrolyte.maxCurrentDensity.Value A/cm^2  alpha=FuelCell.Electrolyte.transferCoefficient.Value  rho_m=FuelCell.Electrolyte.rhoMembrane.Value kg/cm^3  M_m=FuelCell.Electrolyte.mMembrane.Value kg/mol
      settings: InternalSimscapePortConfiguration="{\"Bottom\":[],\"Left\":[{\"id\":\"H\",\"label\":\"H\",\"type\":\"foundation.thermal.thermal\"},{\"id\":\"mdot_w\",\"label\":\"mH20\",\"type\":\"output\"},{\"id\":\"A\",\"label\":\"A\",\"type\":\"GasN.GasN\"},{\"id\":\"mdot_an\",\"label\":\"M_a\",\"type\":\"output\"},{\"id\":\"T_an\",\"label\":\"T_a\",\"type\":\"output\"}],\"Right\":[{\"id\":\"p\",\"label\":\"p\",\"type\":\"foundation.electrical.electrical\"},{\"id\":\"n\",\"label\":\"n\",\"type\":\"foundation.electrical.electrical\"},{\"id\":\"C\",\"label\":\"C\",\"type\":\"GasN.GasN\"},{\"id\":\"mdot_ca\",\"label\":\"M_c\",\"type\":\"output\"},{\"id\":\"T_ca\",\"label\":\"T_c\",\"type\":\"output\"}],\"Top\":[]}"
  Env : GasN_lib/Reservoir (N gas)  p0=FuelCell.CathodeReservoir.p.Value MPa  T0=FuelCell.CathodeReservoir.T.Value degC  constCond=true  comp=GasN.composition_enum.mole  y0=FuelCell.CathodeReservoir.rMoleFractions.Value'  x0=[1; 0; 0; 0]  area=FuelCell.CathodeReservoir.areaPort.Value cm^2
      settings: InternalSimscapePortConfiguration="{\"Bottom\":[],\"Left\":[{\"id\":\"A\",\"label\":\"A\",\"type\":\"GasN.GasN\"}],\"Right\":[],\"Top\":[]}"
  Fcn : Fcn  Expr=0.023*u(1)*u(1)-0.05*u(1)
  Hydrogen Source : Subsystem
  Oxygen Source : Subsystem
  PS-Simulink Converter1 : nesl_utility/PS-Simulink Converter  PhysicalDomain=network_engine_domain  SubClassName=ps_output  LeftPortType=input  RightPortType=output  PseudoPeriodic=off  Frequencies=[]  Unit=Pa  AffineConversion=off
  PowerCalc : Subsystem
  Saturation1 : Saturate  UpperLimit=inf  LowerLimit=0  ZeroCross=off
  Sensor VI : Subsystem
  ThermalMgmt : Subsystem
      mask Display: image('sm_car_vehicle_power_cooling_active1loop_IMAGE.png');
  P_HV : PMIOPort  Side=Right
  N_HV : PMIOPort  Port=2  Side=Right
  P_LV : PMIOPort  Port=3  Side=Right
  N_LV : PMIOPort  Port=4  Side=Right
  Out Bus Element : Outport  PortName=m  Element=i
  Out Bus Element1 : Outport  PortName=m  Element=v
  Out Bus Element2 : Outport  PortName=m  Element=Power
  PBatt : Outport  Port=2
  wires:
  ThermalMgmt/1(PCool) -> PowerCalc/1(PCool)
  Saturation1/1 -> ThermalMgmt/2(Airspeed)
  PS-Simulink Converter1/1 -> Hydrogen Source/2(P_anode)
  Oxygen Source/1(pT) -> [p_comp]
  Oxygen Source/2(Pm) -> PowerCalc/4(Pm)
  Demux/1 -> Out Bus Element1/1, PowerCalc/3(VStack)  "FCV"
  Tcmd/1 -> ThermalMgmt/1(Tcmd)
  PowerCalc/2(PowerBatt) -> PBatt/1
  Fcn/1 -> Saturation1/1
  Sensor VI/1(vi) -> Demux/1
  Demux/2 -> Out Bus Element/1, PowerCalc/2(FCcurr)  "FCcurr"
  VSPD/1 -> Fcn/1
  PowerCalc/1(Power) -> Out Bus Element2/1
  [p_comp] -> Hydrogen Source/1(P_IM)
  Icmd/1 -> Oxygen Source/1(Icmd)
  connections:
  N_HV/RConn1 -- Electrolyte/RConn2 -- Sensor VI/RConn2
  ThermalMgmt/LConn1 -- Electrolyte/LConn1 -- Convection Cathode/RConn1 -- Convection Anode/RConn1
  Cathode Outlet/LConn1 -- Cathode/RConn2
  Electrolyte/LConn3 -- Anode/LConn1
  Oxygen Source/RConn1 -- P_LV/RConn1
  Cathode Inlet/LConn1 -- Oxygen Source/LConn1
  Cathode Outlet/RConn1 -- Env/LConn1
  Electrolyte/LConn5 -- Anode/LConn3
  Electrolyte/RConn5 -- Cathode/LConn3
  Hydrogen Source/RConn1 -- Anode Inlet/LConn1
  Oxygen Source/RConn2 -- N_LV/RConn1
  PS-Simulink Converter1/LConn1 -- Anode/RConn3
  Electrolyte/RConn4 -- Cathode/LConn2
  Electrolyte/LConn4 -- Anode/LConn2
  Anode Inlet/RConn1 -- Anode/RConn1
  Cathode Inlet/RConn1 -- Cathode/RConn1
  Sensor VI/RConn1 -- P_HV/RConn1
  Electrolyte/RConn1 -- Sensor VI/LConn1
  Electrolyte/RConn3 -- Cathode/LConn1
  Convection Cathode/LConn1 -- Cathode/LConn4
  Convection Anode/LConn1 -- Anode/LConn4
  Cap/LConn1 -- Anode/RConn2

== system Power_FuelCell1Motor/FuelCell1Motor/Fuel Cell/Thermal ==
  Controlled Heat Flow Rate Source : fl_lib/Thermal/Thermal Sources/Controlled Heat Flow Rate Source
      settings: SourceProductName=Simscape
  PS Gain : fl_lib/Physical Signals/Functions/PS Gain  Commented=on  gain=FuelCell.Converter.resistance.Value Ohm
  PS Math Function : fl_lib/Physical Signals/Functions/PS Math Function  Commented=on  fcn_choice=foundation.enum.math_function.square
      settings: SourceProductName=Simscape  SourceProductBaseCode=SS
  PS Power Function : customMath_lib/PS Power Function  resistance=FuelCell.Converter.resistance.Value Ohm
      settings: InternalSimscapePortConfiguration="{\"Bottom\":[],\"Left\":[{\"id\":\"I\",\"label\":\"\",\"type\":\"input\"}],\"Right\":[{\"id\":\"O\",\"label\":\"\",\"type\":\"output\"}],\"Top\":[]}"
  Thermal Mass : fl_lib/Thermal/Thermal Elements/Thermal Mass  mass=FuelCell.Converter.mThermal.Value kg  sp_heat=FuelCell.Converter.Cp.Value J/kg/K  T_specify=off  T_priority=High  T=300 K  T_nominal_specify=off  T_nominal_unit=K  T_nominal_value=1  Q_specify=off  Q_priority=None  Q=0 W  Q_nominal_specify=off  Q_nominal_unit=W  Q_nominal_value=1
  Thermal Resistance : fl_lib/Thermal/Thermal Elements/Thermal Resistance  resistance=FuelCell.Converter.rConvection.Value K/W  T_specify=off  T_priority=None  T=0 K  T_nominal_specify=off  T_nominal_unit=K  T_nominal_value=1  Q_specify=off  Q_priority=None  Q=0 W  Q_nominal_specify=off  Q_nominal_unit=W  Q_nominal_value=1
      settings: SourceProductName=Simscape  SourceProductBaseCode=SS
  Thermal Reference2 : fl_lib/Thermal/Thermal Elements/Thermal Reference
  H : PMIOPort  Side=Right
  i : PMIOPort  Port=2  Side=Left
  connections:
  PS Power Function/RConn1 -- Controlled Heat Flow Rate Source/RConn1
  PS Math Function/RConn1 -- PS Gain/LConn1
  Thermal Resistance/LConn1 -- Thermal Mass/LConn1 -- Controlled Heat Flow Rate Source/LConn1
  Thermal Reference2/LConn1 -- Controlled Heat Flow Rate Source/RConn2
  PS Power Function/LConn1 -- i/RConn1
  H/RConn1 -- Thermal Resistance/RConn1

== system Power_FuelCell1Motor/FuelCell1Motor/Motor/Sensing Current ==
  Current Sensor : fl_lib/Electrical/Electrical Sensors/Current Sensor
  PS-Simulink Converter : nesl_utility/PS-Simulink Converter  PhysicalDomain=network_engine_domain  SubClassName=ps_output  LeftPortType=input  RightPortType=output  PseudoPeriodic=off  Frequencies=[]  Unit=A  AffineConversion=off
  + : PMIOPort  Side=Right
  - : PMIOPort  Port=2  Side=Left
  i : Outport
  wires:
  PS-Simulink Converter/1 -> i/1
  connections:
  PS-Simulink Converter/LConn1 -- Current Sensor/RConn1
  Current Sensor/LConn1 -- +/RConn1
  Current Sensor/RConn2 -- -/RConn1

== system Power_FuelCell1Motor/FuelCell1Motor/Motor/Sensing Torque ==
  PS-Simulink Converter : nesl_utility/PS-Simulink Converter  PhysicalDomain=network_engine_domain  SubClassName=ps_output  LeftPortType=input  RightPortType=output  PseudoPeriodic=off  Frequencies=[]  Unit=N*m  AffineConversion=off
  Torque Sensor : fl_lib/Mechanical/Mechanical Sensors/Ideal Torque Sensor
  C : PMIOPort  Side=Right
  R : PMIOPort  Port=2  Side=Left
  trq : Outport
  wires:
  PS-Simulink Converter/1 -> trq/1
  connections:
  Torque Sensor/RConn2 -- PS-Simulink Converter/LConn1
  Torque Sensor/RConn1 -- C/RConn1
  Torque Sensor/LConn1 -- R/RConn1

== system Power_FuelCell1Motor/FuelCell1Motor/Thermal System/Pump Control ==
  TAmb : Inport
  TMotor : Inport  Port=2
  Add : Sum  Inputs=|-+
  PID Controller : simulink/Continuous/PID Controller  Controller=PI  Form=Parallel  TimeDomain=Continuous-time  SampleTime=-1  IntegratorMethod=Forward Euler  FilterMethod=Forward Euler  ControllerParametersSource=internal  P=Cooling.Control.Kp.Value  I=Cooling.Control.Ki.Value  D=0  UseFilter=on  N=100  TunerSelectOption=Transfer Function Based (PID Tuner App)  ZeroCross=off  InitialConditionSource=internal  InitialConditionForIntegrator=0  InitialConditionForFilter=0  DifferentiatorICPrevScaledInput=0  ExternalReset=none  TrackingMode=off  Kt=1  LimitOutput=on  UpperSaturationLimit=0.1  LowerSaturationLimit=0  LinearizeAsGain=on  AntiWindupMode=none  Kb=1  POutMin=[]  POutMax=[]  IOutMin=[]  IOutMax=[]  DOutMin=[]  DOutMax=[]  NOutMin=[]  NOutMax=[]  SumOutMin=[]  SumOutMax=[]  SaturationOutMin=[]  SaturationOutMax=[]  PParamMin=[]  PParamMax=[]  IParamMin=[]  IParamMax=[]  DParamMin=[]  DParamMax=[]  NParamMin=[]  NParamMax=[]  KbParamMin=[]  KbParamMax=[]  KtParamMin=[]  KtParamMax=[]  KbOutMin=[]  KbOutMax=[]  KtOutMin=[]  KtOutMax=[]  IntegratorOutMin=[]  IntegratorOutMax=[]  FilterOutMin=[]  FilterOutMax=[]  SumI1OutMin=[]  SumI1OutMax=[]  SumI2OutMin=[]  SumI2OutMax=[]  SumI3OutMin=[]  SumI3OutMax=[]  SumI4OutMin=[]  SumI4OutMax=[]  SumDOutMin=[]  SumDOutMax=[]  DifferentiatorOutMin=[]  DifferentiatorOutMax=[]  FilterDiffOutCoefMin=[]  FilterDiffOutCoefMax=[]  ReciprocalOutMin=[]  ReciprocalOutMax=[]  SumDenOutMin=[]  SumDenOutMax=[]  SumNumOutMin=[]  SumNumOutMax=[]  DivideOutMin=[]  DivideOutMax=[]  IntegratorContinuousStateAttributes=''  IntegratorStateMustResolveToSignalObject=off  IntegratorRTWStateStorageClass=Auto  FilterContinuousStateAttributes=''  FilterStateMustResolveToSignalObject=off  FilterRTWStateStorageClass=Auto  ParallelPVariant=InternalParameters  IdealPVariant=Disabled  IVariant=InternalParameters  DVariant=Disabled  IntegratorVariant=Continuous  SatVariant=Enabled  AWVariant=Passthrough  PCopyVariant=Disabled  TRVariant=Disabled  FdbkBlocksVariant=Forward  IdealPFdbkVariant=Disabled  SatFdbkVariant=Disabled  DerivativeFilterVariant=Disabled  NVariant=Disabled  NCopyVariant=Disabled_SignalSpec  FilterICVariant=Disabled  IntegratorICVariant=InternalICs  ExternalResetVariant=Disabled  TRSumVariant=Passthrough  SumFdbkVariant=Disabled  SumVariant=Sum_PI
  Transfer Fcn : TransferFcn  Denominator=[0.1 1]
  Pump_flw : Outport
  wires:
  Add/1 -> PID Controller/1
  PID Controller/1 -> Transfer Fcn/1  "Pump_flw"
  TAmb/1 -> Add/1
  TMotor/1 -> Add/2
  Transfer Fcn/1 -> Pump_flw/1

== system Power_FuelCell1Motor/FuelCell1Motor/Thermal System/Sensing T Amb ==
  PS-Simulink Converter1 : nesl_utility/PS-Simulink Converter  PhysicalDomain=network_engine_domain  SubClassName=ps_output  LeftPortType=input  RightPortType=output  PseudoPeriodic=off  Frequencies=[]  Unit=K  AffineConversion=off
  Temperature Sensor : fl_lib/Thermal/Thermal Sensors/Temperature Sensor
  Thermal Reference : fl_lib/Thermal/Thermal Elements/Thermal Reference
  A : PMIOPort  Side=Left
  T : Outport
  wires:
  PS-Simulink Converter1/1 -> T/1
  connections:
  Temperature Sensor/LConn1 -- A/RConn1
  Temperature Sensor/RConn2 -- PS-Simulink Converter1/LConn1
  Temperature Sensor/RConn1 -- Thermal Reference/LConn1

== system Power_FuelCell1Motor/FuelCell1Motor/Thermal System/Sensing T Conv ==
  PS-Simulink Converter1 : nesl_utility/PS-Simulink Converter  PhysicalDomain=network_engine_domain  SubClassName=ps_output  LeftPortType=input  RightPortType=output  PseudoPeriodic=off  Frequencies=[]  Unit=K  AffineConversion=off
  Temperature Sensor : fl_lib/Thermal/Thermal Sensors/Temperature Sensor
  Thermal Reference : fl_lib/Thermal/Thermal Elements/Thermal Reference
  A : PMIOPort  Side=Left
  T : Outport
  wires:
  PS-Simulink Converter1/1 -> T/1
  connections:
  Temperature Sensor/LConn1 -- A/RConn1
  Temperature Sensor/RConn2 -- PS-Simulink Converter1/LConn1
  Temperature Sensor/RConn1 -- Thermal Reference/LConn1

== system Power_FuelCell1Motor/FuelCell1Motor/Thermal System/Sensing T MotorR ==
  PS-Simulink Converter1 : nesl_utility/PS-Simulink Converter  PhysicalDomain=network_engine_domain  SubClassName=ps_output  LeftPortType=input  RightPortType=output  PseudoPeriodic=off  Frequencies=[]  Unit=K  AffineConversion=off
  Temperature Sensor : fl_lib/Thermal/Thermal Sensors/Temperature Sensor
  Thermal Reference : fl_lib/Thermal/Thermal Elements/Thermal Reference
  A : PMIOPort  Side=Left
  T : Outport
  wires:
  PS-Simulink Converter1/1 -> T/1
  connections:
  Temperature Sensor/RConn1 -- Thermal Reference/LConn1
  Temperature Sensor/RConn2 -- PS-Simulink Converter1/LConn1
  Temperature Sensor/LConn1 -- A/RConn1
